simulink model "proje_p_1"  (R2016a)
settings: Solver=VariableStepAuto  StartTime=0.0  StopTime=40  RelTol=1e-3
undefined symbols (not defined in the file or in its folder): j
libraries: powerlib x8
settings Model: Creator=acer  LastModifiedBy=gunge

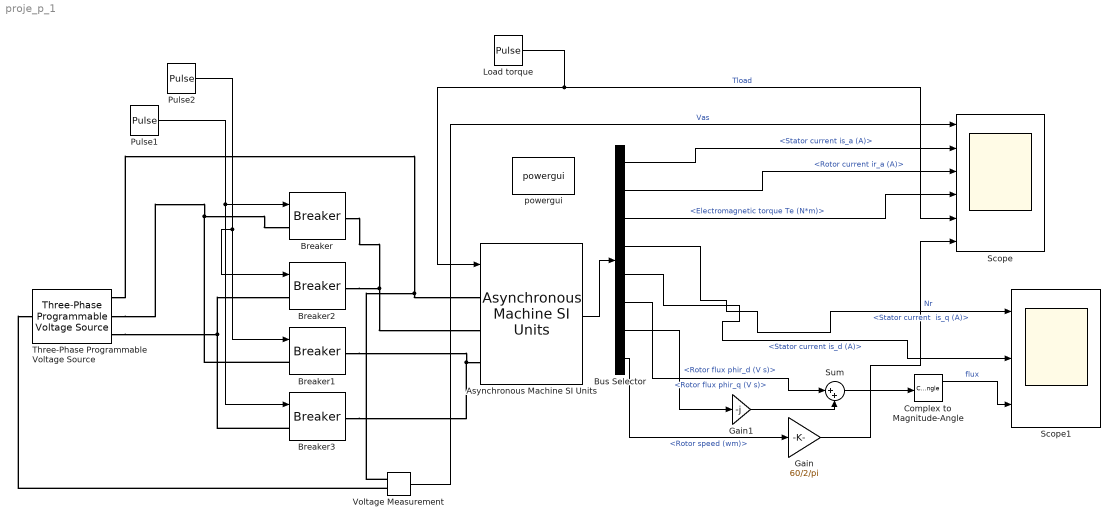
== system proje_p_1 ==
  Asynchronous Machine SI Units : powerlib/Machines/Asynchronous Machine SI Units  RotorType=Squirrel-cage  PresetModel=No  MechanicalLoad=Torque Tm  ShowDetailedParameters=on  ReferenceFrame=Rotor  Units=SI  MeasurementBus=off  NominalParameters=[3730 230 60]  Stator=[0.531 0.00252]  Rotor=[0.408 0.00252]  Cage1=[0.4155 0.002066]  Cage2=[0.4168 0.0003495]  Lm=0.0847  Mechanical=[1.1 0 2]  PolePairs=2  InitialConditions=[1 0 0 0 0 0 0 0]  SimulateSaturation=off  Saturation=[14.03593122, 27.81365428, 53.79336849, 72.68890987, 97.98006896, 148.6815601, 215.7428561, 302.9841135, 428.7778367 ; 230, 322, 414, 460, 506, 552, 598, 644, 690]  LoadFlowParameters=1492000  TsPowergui=0  TsBlock=-1  IterativeModel=Trapezoidal non iterative  IterativeDiscreteModel=Trapezoidal non iterative  Pmec=1.492e+006
  Breaker{,1..3} (4 alike) : powerlib/Elements/Breaker  InitialState=0  SwitchingTimes="[1/60  5/60]"  External=on  BreakerResistance=0.01  SnubberResistance=1e6  SnubberCapacitance=inf  Measurements=None  MoreParameters=on  NoBreakLoop=off
  Bus Selector : BusSelector  OutputSignals="Stator measurements.Stator current is_a (A),Rotor measurements.Rotor current ir_a (A),Mechanical.Electromagnetic torque Te (N*m),Stator measurements.Stator current  is_q (A),Stator measurements.Stator current is_d (A),Rotor measurements.Rotor flux phir_q (V s),Rotor measurements.Rotor flux phir_d (V s),Mechanical.Rotor speed (wm)"
  Complex to Magnitude-Angle : ComplexToMagnitudeAngle
  Gain : Gain  Gain=60/2/pi
  Gain1 : Gain  Gain=-j
  Load torque : DiscretePulseGenerator  PulseType=Time based  Amplitude=10  Period=40  PulseWidth=55  PhaseDelay=10
  Pulse1 : DiscretePulseGenerator  PulseType=Time based  Amplitude=15  Period=40  PulseWidth=37.5
  Pulse2 : DiscretePulseGenerator  PulseType=Time based  Amplitude=5  Period=40  PulseWidth=62.5  PhaseDelay=15
  Scope : Scope  NumInputPorts=6
  Scope1 : Scope  NumInputPorts=3
  Sum : Sum  Inputs=|++
  Three-Phase Programmable Voltage Source : powerlib/Electrical Sources/Three-Phase Programmable Voltage Source  PositiveSequence="[230  0 60]"  VariationEntity=None  VariationType=Table of time-amplitude pairs  VariationTypeAlt=Step  VariationStep=0.5  VariationRate=10  VariationMagnitude=0.3  VariationFrequency=2  VariationTiming=[1 2]  VariationPhaseA=off  Amplitudes=[1 0.8 1.2 1.0]  TimeValues=[0 0.1 0.15 0.2]  HarmonicGeneration=off  HarmonicA=[3 0.2 -25 0]  HarmonicB=[2 0.15 35 2]  Timing="[0.05  3]"  BusType=swing  Pref=0  Qref=0  Qmin=-inf  Qmax=inf
  Voltage Measurement : powerlib/Measurements/Voltage Measurement  PhasorSimulation=off  OutputType=Complex  PSBequivalent=0
  powergui : powerlib/powergui  Priority=1  SimulationMode=Discrete  SolverType=Tustin/Backward Euler (TBE)  SampleTime=10e-6  frequency=60  SPID=off  DisableSnubberDevices=off  DisableRonSwitches=off  DisableVfSwitches=off  SwTol=0  DisplayEquations=off  Interpol=off  ExternalGateDelay=off  methode=off  Ts=10  FunctionMessages=off  echomessages=off  HookPort=off  EnableUseOfTLC=off  x0status=blocks  frequencyindice=60  Pbase=100e6  ErrMax=1e-4  Iterations=50  UnitsV=kV  UnitsW=MW  buscounter=0  RestoreLinks=warning  ResistiveCurrentMeasurement=off  Frange=[0:2:500]  Ylog=off  Xlog=on  ShowGrid=off  save=off  variable=ZData  structure=0  ZoomFFT=off  StartTime=0.0  cycles=1  DisplayStyle=1  fundamental=60  FreqAxis=off  MaxFrequency=1000  frequencyindicesteady=1  RmsSteady=1  display=off
  wires:
  Asynchronous Machine SI Units/1 -> Bus Selector/1
  Voltage Measurement/1 -> Scope/1  "Vas"
  Bus Selector/1 -> Scope/2  "<Stator current is_a (A)>"
  Bus Selector/2 -> Scope/3  "<Rotor current ir_a (A)>"
  Bus Selector/3 -> Scope/4  "<Electromagnetic torque Te (N*m)>"
  Load torque/1 -> Scope/5, Asynchronous Machine SI Units/1  "Tload"
  Bus Selector/8 -> Gain/1  "<Rotor speed (wm)>"
  Gain/1 -> Scope/6  "Nr"
  Pulse1/1 -> Breaker3/1, Breaker/1
  Pulse2/1 -> Breaker1/1, Breaker2/1
  Bus Selector/4 -> Scope1/1  "<Stator current  is_q (A)>"
  Bus Selector/5 -> Scope1/2  "<Stator current is_d (A)>"
  Bus Selector/7 -> Gain1/1  "<Rotor flux phir_d (V s)>"
  Bus Selector/6 -> Sum/1  "<Rotor flux phir_q (V s)>"
  Gain1/1 -> Sum/2
  Sum/1 -> Complex to Magnitude-Angle/1
  Complex to Magnitude-Angle/1 -> Scope1/3  "flux"
  connections:
  Three-Phase Programmable Voltage Source/RConn1 -- Voltage Measurement/LConn1 -- Asynchronous Machine SI Units/LConn1
  Voltage Measurement/LConn2 -- Three-Phase Programmable Voltage Source/LConn1
  Three-Phase Programmable Voltage Source/RConn2 -- Breaker1/LConn1 -- Breaker/LConn1
  Breaker/RConn1 -- Breaker2/RConn1 -- Asynchronous Machine SI Units/LConn2
  Three-Phase Programmable Voltage Source/RConn3 -- Breaker2/LConn1 -- Breaker3/LConn1
  Breaker1/RConn1 -- Breaker3/RConn1 -- Asynchronous Machine SI Units/LConn3
